simulink library "Constant_Power_Source"  (R2018b)
settings: Solver=VariableStepAuto  StartTime=0.0  StopTime=10.0  RelTol=1e-3
settings Model: Creator=ga69qig  LastModifiedBy=ga69qig
settings SFSimCC: SimUseLocalCustomCode=off
settings RTWCC: RTWUseLocalCustomCode=off

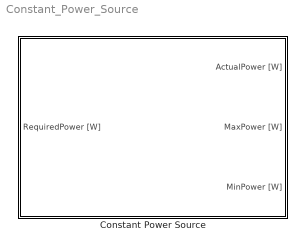
== system Constant_Power_Source ==
  Constant Power Source : Subsystem  mask(SB){MaxPower=400000, MinPower=-10000, LocalSampleTime=-1}
      mask prompts: MaxPower "Maximum Power [W]"; MinPower "Minimum Power [W]"; LocalSampleTime "Local System Sample-Time [s]"
      mask help:
      | <Author> Benedikt Danquah</Author>
      | <Date> 01/2019 </Date>
      |
      | <Description>
      | The model outputs the custom input of the maximal/minimal power. The required power is compared to the custom input of the max./min. power and, if necessary, saturated.
      | </Description>
      mask init:
      | GlobalSampleTime = CalcGlobalSampleTime(LocalSampleTime);
      mask Help:
      | <Parameters>
      | Maximum Power [W]
      | Minimum Power [W]
      | </Parameters>
      | 
      | <Inputs>
      | RequiredPower [W]
      | 	<sign orientation> [+] discharge </sign orientation>
      | </Inputs>
      | 
      | <Outputs>
      | ActualPower [W]
      | 	<sign orientation> [+] discharge </sign orientation>
      | MaxPower [W]
      | MinPower [W]
      | </Outputs>
      mask TypeOptions LocalSampleTime: RequiredPower [W]/SampleTime
      mask DialogControl Container3 Prompt: Documentation:
      mask DialogControl Control2 Prompt: %<MaskHelp>
      mask DialogControl Container8 Prompt: Sample Time
      mask Display:
      | [picturexpos,pictureypos,picturewidth,pictureheight] = ...
      |     CalcBlockPicturePosition(gcb,0.5,0.01,0.1,100,100); % calculating picture position depending on Block size and minimum margin size
      | image('Constant_Power_Source.svg',[picturexpos pictureypos picturewidth pictureheight]) % plot picture to block

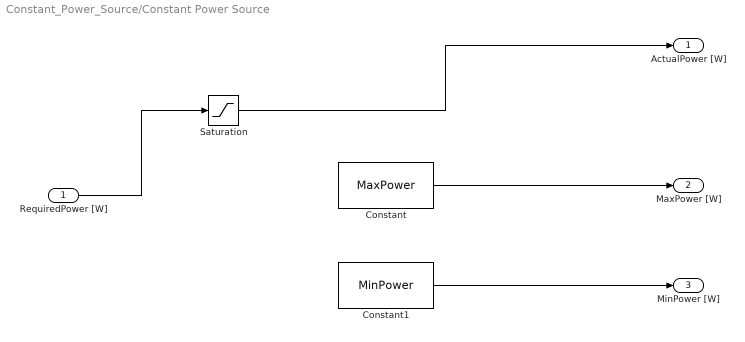
== system Constant_Power_Source/Constant Power Source ==
  RequiredPower [W] : Inport  SampleTime=LocalSampleTime
  Constant : Constant  Value=MaxPower
  Constant1 : Constant  Value=MinPower
  Saturation : Saturate  UpperLimit=MaxPower  LowerLimit=MinPower
  ActualPower [W] : Outport  SampleTime=GlobalSampleTime
  MaxPower [W] : Outport  Port=2  SampleTime=GlobalSampleTime
  MinPower [W] : Outport  Port=3  SampleTime=GlobalSampleTime
  wires:
  Constant/1 -> MaxPower [W]/1
  Constant1/1 -> MinPower [W]/1
  Saturation/1 -> ActualPower [W]/1
  RequiredPower [W]/1 -> Saturation/1
